simulink model "Main"  (R2021a)
settings: Solver=FixedStepDiscrete  StartTime=0.0  StopTime=3600  RelTol=1e-3  EnableMultiTasking=on
model workspace (MAT data in the model file):
  Rp_LUT = [0.0013213692114; 0.00132154036622; 0.00132170974574; 0.00132196270497; 0.00132238459891; 0.00132306078259; 0.001324076611; 0.00132551743918; 0.00132746862213; 0.00133001551485; 0.00133324347238; 0.00133723784971; 0.00134208400186; 0.00134786728385; 0.00135467305069; 0.00136258665738; 0.00137169345895; 0.0013820788104; 0.00139382806676; 0.00140702658302; 0.00142175971421; 0.00143811281533; 0.00145617124141; 0.00147602034745; 0.00149774548846; 0.00152143201947; 0.00154716529547; 0.00157503067149; 0.00160511350254; 0.00163749914362; 0.00167227294976; 0.00170952027597; 0.00174932647725]
  Rs_LUT = [0.00434482474387; 0.00419789131326; 0.00406794421213; 0.00395261023619; 0.00384993859762; 0.00375831094443; 0.00367637344064; 0.00360298484472; 0.00353717635596; 0.00347812023039; 0.00342510501023; 0.00337751579607; 0.00333481840341; 0.00329654653965; 0.00326229135038; 0.00323169283953; 0.0032044327828; 0.00318022883979; 0.00315882963473; 0.00314001062482; 0.00312357061298; 0.00310932879063; 0.00309712221887; 0.00308680367416; 0.00307823979817; 0.00307130950314; 0.00306590259229; 0.0030619185623; 0.00305926556038; 0.00305785947318; 0.00305762312844; 0.00305848559347; 0.00306038155708]
  ocv_LUT = [2.99933110368 3.09522958218 3.19229911251 3.28822862042 3.38021163392 3.46527495221 3.54075046741 3.60476472978 3.6565797805 3.69666389655 3.72648450624 3.74812569713 3.76387527119 3.77589456216 3.78601862589 3.79567838914 3.8059086629 3.81740274636 3.8305836234 3.84567360605 3.86275382653 3.88181106067 3.90277255901 3.92553086689 3.94996087864 3.97593115245 4.00331113101 4.03197552137 4.06180675196 4.09269615923 4.12454435791 4.15726110493 4.19076486521]
  soc_LUT = [0 0.03125 0.0625 0.09375 0.125 0.15625 0.1875 0.21875 0.25 0.28125 0.3125 0.34375 0.375 0.40625 0.4375 0.46875 0.5 0.53125 0.5625 0.59375 0.625 0.65625 0.6875 0.71875 0.75 0.78125 0.8125 0.84375 0.875 0.90625 0.9375 0.96875 1]
  tau_LUT = [1017.78463693; 1013.76600608; 1009.7449439; 1005.78640776; 1001.95428754; 998.311501769; 994.921511879; 991.866028712; 989.396935472; 988.873758798; 996.773296442; 1035.63338161; 1158.31056663; 1435.4479506; 1876.25610659; 2330.74386132; 2537.63289906; 2355.40456965; 1912.97681891; 1471.93759841; 1191.35445849; 1068.59098544; 1033.79837309; 1032.53037298; 1041.04700517; 1052.45769279; 1065.37076923; 1079.60983832; 1095.18901085; 1112.14336121; 1130.50876964; 1150.32016376; 1171.6114047]
values from neighbouring files (symbols this model uses):
  Ts = 0.2    [Parameters.m]
libraries: fl_lib x4, nesl_utility x4, ee_lib x1, sharedTrackingLibrary x1
settings Model: SimulationMode=accelerator  OrderedModelArguments=off  Creator=oscar  LastModifiedBy=oscar
settings SolverCC: AutoInsertRateTranBlk=on
settings DataIOCC: SaveOutput=off  SaveTime=off
settings OptimizationCC: DefaultParameterBehavior=Inlined  InlineInvariantSignals=on  EnhancedBackFolding=on  PassReuseOutputArgsAs=Individual arguments  StateBitsets=on  DataBitsets=on  ZeroExternalMemoryAtStartup=off  ZeroInternalMemoryAtStartup=off  NoFixptDivByZeroProtection=on  LifeSpan=1  OptimizeBlockOrder=speed  DifferentSizesBufferReuse=on  EfficientTunableParamExpr=on
settings DebuggingCC: ParameterTunabilityLossMsg=error
settings HardwareCC: ProdBitPerPointer=32  ProdBitPerSizeT=32  ProdBitPerPtrDiffT=32  ProdLargestAtomicInteger=Long  ProdLargestAtomicFloat=Double  ProdWordSize=32  ProdHWDeviceType=ARM Compatible->ARM Cortex-M
settings SFSimCC: MATLABDynamicMemAlloc=off
settings RTWCC: SystemTargetFile=ert.tlc  TLCOptions=-p0  GenCodeOnly=on  TemplateMakefile=ert_default_tmf  GenerateReport=on  RTWVerbose=off  IncludeHyperlinkInReport=on  LaunchReport=on
settings CodeAppCC: ForceParamTrailComments=on  IgnoreCustomStorageClasses=off  OperatorAnnotations=on  SimulinkDataObjDesc=on  SFDataObjDesc=on  CustomSymbolStrGlobalVar=rt$N$M  CustomSymbolStrType=$N$M  CustomSymbolStrFcn=$N$M$F  CustomSymbolStrMacro=$N$M  InsertBlockDesc=on
settings ERTTargetCC: TargetLangStandard=C99 (ISO)  CodeReplacementLibrary=ISO_C  GenerateSampleERTMain=on  IncludeMdlTerminateFcn=off  SuppressErrorStatus=on  SupportAbsoluteTime=off  SupportNonFinite=off  SupportComplex=off  InlinedParameterPlacement=NonHierarchical  RootIOFormat=Structure reference  ERTCustomFileTemplate=example_file_process.tlc
settings SimscapeCC: SimscapeLogType=all  SimscapeLogOpenViewer=on  SimscapeLogLimitData=off

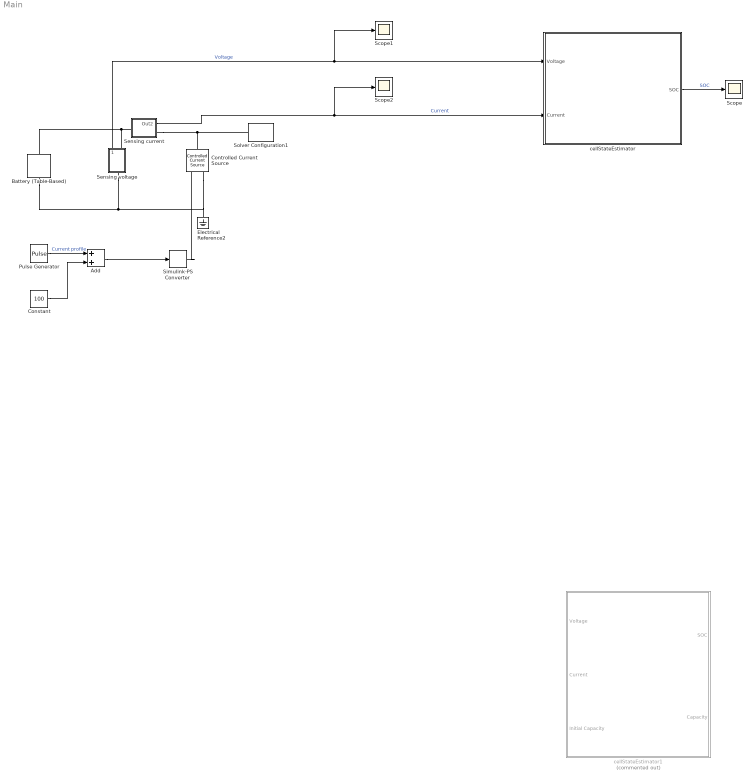
== system Main ==
  Add : Sum
  Battery (Table-Based) : ee_lib/Sources/Battery (Table-Based)  SOC_vec=soc_LUT  T_dependence=ee.enum.temperature_dependence.no  prm_dir=ee.enum.battery.prm_dir.noCurrentDirectionality  T_vec=[273.15, 298.15, 323.15] K  V0_mat=[3.2, 3.1, 3.14; 3.25, 3.27, 3.3; 3.28, 3.31, 3.34; 3.33, 3.5, 3.59] V  V0_vec=ocv_LUT V  R0_mat=[.03, .015, .002; .04, .017, .008; .039, .012, .006; .027, .013, .021] Ohm  R0_vec=Rs_LUT Ohm  R0_dis_mat=[.03, .015, .002; .04, .017, .008; .039, .012, .006; .027, .013, .021] Ohm  R0_dis_vec=[.015, .017, .012, .013] Ohm  R0_ch_mat=[.03, .015, .002; .04, .017, .008; .039, .012, .006; .027, .013, .021] Ohm  R0_ch_vec=[.015, .017, .012, .013] Ohm  AH_vec=[2.9, 4.1, 4.2] hr*A  AH=C hr*A  prm_leak=ee.enum.battery.prm_leak.disabled  Rleak_vec=[8000, 7000, 6000] Ohm  Rleak=7e3 Ohm  extrapolation_option=ee.enum.extrapolation.linear  prm_dyn=ee.enum.battery.prm_dyn.rc1  R1_mat=[.089, .076, .01; .042, .022, .099; .019, .007, .002; .051, .043, .029] Ohm  R1_vec=Rp_LUT Ohm  tau1_mat=[44, 148, 235; 93, 110, 1000; 19, 27, 133; .5, 22, 3] s  tau1_vec=tau_LUT s  R2_mat=[.014, .382, .407; .028, .006, .007; .014, .007, .006; .333, .956, .912] Ohm  R2_vec=[.382, .006, .007, .956] Ohm  tau2_mat=[1, 44, 5644; 11, 24, 506; 2, 14, 330; 3310, 13419, 30216] s  tau2_vec=[44, 24, 14, 13419] s  R3_mat=[.014, .382, .407; .028, .006, .007; .014, .007, .006; .333, .956, .912] Ohm  R3_vec=[.382, .006, .007, .956] Ohm  tau3_mat=[1, 44, 5644; 11, 24, 506; 2, 14, 330; 3310, 13419, 30216] s  tau3_vec=[44, 24, 14, 13419] s  R4_mat=[.014, .382, .407; .028, .006, .007; .014, .007, .006; .333, .956, .912] Ohm  R4_vec=[.382, .006, .007, .956] Ohm  tau4_mat=[1, 44, 5644; 11, 24, 506; 2, 14, 330; 3310, 13419, 30216] s  tau4_vec=[44, 24, 14, 13419] s  R5_mat=[.014, .382, .407; .028, .006, .007; .014, .007, .006; .333, .956, .912] Ohm  R5_vec=[.382, .006, .007, .956] Ohm  tau5_mat=[1, 44, 5644; 11, 24, 506; 2, 14, 330; 3310, 13419, 30216] s  tau5_vec=[44, 24, 14, 13419] s  prm_fade=ee.enum.battery.prm_fade.equations  N0=10  dV0=0  dR0=0  dAH=-2  dRleak=0  dR1=0  dR2=0  dR3=0  dR4=0  dR5=0  N0vec=[100, 200, 300]  Tfadevec=[298.15, 323.15] K  dV0vec=[0, 0, 0]  dR0vec=[0, 0, 0]  dAHvec=[0, 0, 0]  dRleakvec=[0, 0, 0]  dR1vec=[0, 0, 0]  dR2vec=[0, 0, 0]  dR3vec=[0, 0, 0]  dR4vec=[0, 0, 0]  dR5vec=[0, 0, 0]  dV0mat=[0, 0; 0, 0; 0, 0]  dR0mat=[0, 0; 0, 0; 0, 0]  dAHmat=[0, 0; 0, 0; 0, 0]  dRleakmat=[0, 0; 0, 0; 0, 0]  dR1mat=[0, 0; 0, 0; 0, 0]  dR2mat=[0, 0; 0, 0; 0, 0]  dR3mat=[0, 0; 0, 0; 0, 0]  dR4mat=[0, 0; 0, 0; 0, 0]  dR5mat=[0, 0; 0, 0; 0, 0]  prm_age=ee.enum.battery.prm_age.disabled  prm_age_OCV=ee.enum.battery.prm_age_OCV.OCV  OCV_age=0.9  SOC_age=0.6  storage_dt_age_vec=[0] d  storage_T_age_vec=[273] K  OCV_scaling_age=2.2134e6  OCV_offset_age=1.632e6  temp_exp_age=0.515833569 V  t_exp_age=0.75  T_age_vec=[273.15, 298.15, 323.15] K  dt_age_vec=[90, 180, 270, 360] d  dR0_age_vec=[0, 0, 0]  t_meas_dR0_age=100 d  dR0_age_mat=[0, 0, 0; 0, 0, 0; 0, 0, 0; 0, 0, 0]  temperature=298.15 K  i_specify=off  i_priority=None  i=0 A  i_nominal_specify=off  i_nominal_unit=A  i_nominal_value=1  v_specify=off  v_priority=None  v=0 V  v_nominal_specify=off  v_nominal_unit=V  v_nominal_value=1  stateOfCharge_specify=on  stateOfCharge_priority=High  stateOfCharge=0.7  stateOfCharge_nominal_specify=off  stateOfCharge_nominal_unit=1  stateOfCharge_nominal_value=1  num_cycles_specify=off  num_cycles_priority=High  num_cycles=0  num_cycles_nominal_specify=off  num_cycles_nominal_unit=1  num_cycles_nominal_value=1  thermal_mass=30000 J/K  temperature_specify=off  temperature_priority=High  temperature_nominal_specify=off  temperature_nominal_unit=K  temperature_nominal_value=1
      settings: SourceProductBaseCode=PS  InternalSimscapePortConfiguration="{\"Bottom\":[],\"Left\":[{\"id\":\"p\",\"label\":\"+\",\"type\":\"foundation.electrical.electrical\"}],\"Right\":[{\"id\":\"n\",\"label\":\"-\",\"type\":\"foundation.electrical.electrical\"}],\"Top\":[]}"
  Constant : Constant  Value=100
  Controlled Current Source : fl_lib/Electrical/Electrical Sources/Controlled Current Source
  Electrical Reference2 : fl_lib/Electrical/Electrical Elements/Electrical Reference
  Pulse Generator : DiscretePulseGenerator  Amplitude=-200  Period=30/0.2  PulseWidth=0.5*30/0.2  SampleTime=0.2
  Scope : Scope
  Scope1 : Scope
  Scope2 : Scope
  Sensing current : Subsystem
      mask Display: disp('i')
  Sensing voltage : Subsystem
      mask Display: disp('i')
  Simulink-PS Converter : nesl_utility/Simulink-PS Converter  PhysicalDomain=network_engine_domain  SubClassName=ps_input  LeftPortType=input  RightPortType=output  PseudoPeriodic=off  Frequencies=[]  NoiseDistribution=none  NoiseParameters=[]  Unit=A  AffineConversion=off  FilteringAndDerivatives=zero  SimscapeFilterOrder=1  InputFilterTimeConstant=0.001  UdotUserProvided=1
      settings: SourceProductBaseCode=PW,SS
  Solver Configuration1 : nesl_utility/Solver Configuration  PhysicalDomain=network_engine_domain  SubClassName=solver  LeftPortType=input  RightPortType=generic  Tones=[]  Harmonics=[]  SimulateNoise=off  Profile=off  UseLocalSampling=off  EnableSwitchedLinearOptims=on  FrequencyDomain=off  UseCCode=off  RelTol=0.001  AbsTol=1e-06  MinStep=1e-09  ToWorkspace=off  RevertToSquareIcSolve=off  NumHomotopyIterations=100  PhasorMode=off  PhasorModeNumHarmonics=1  DoDC=off  ResidualTolerance=1e-09  UseLocalSolver=on  LocalSolverChoice=NE_BACKWARD_EULER_ADVANCER  LocalSolverSampleTime=Ts  DoFixedCost=on  MaxNonlinIter=3  MaxModeIter=2  ComputeImpulses=off  ImpulseIterations=2  LinearAlgebra=auto  EquationFormulation=NE_TIME_EF  DelaysMemoryBudget=1024  AutomaticFiltering=on  FilteringTimeConstant=0.001  PartitionStorageMethod=AS_NEEDED  PartitionMemoryBudget=1024  PartitionMethod=FAST
      settings: SourceProductBaseCode=PW,SS
  cellStateEstimator : Subsystem
  cellStateEstimator1 : Subsystem  Commented=on
  wires:
  cellStateEstimator/1(SOC) -> Scope/1  "SOC"
  Sensing voltage/1(Out1) -> Scope1/1, cellStateEstimator/1(Voltage)  "Voltage"
  Pulse Generator/1 -> Add/1  "Current profile"
  Sensing current/1(Out2) -> Scope2/1, cellStateEstimator/2(Current)  "Current"
  Constant/1 -> Add/2
  Add/1 -> Simulink-PS Converter/1
  connections:
  Sensing voltage/RConn1 -- Battery (Table-Based)/LConn1 -- Sensing current/LConn1
  Solver Configuration1/RConn1 -- Sensing current/RConn1 -- Controlled Current Source/LConn1
  Electrical Reference2/LConn1 -- Controlled Current Source/RConn2 -- Battery (Table-Based)/RConn1 -- Sensing voltage/LConn1
  Simulink-PS Converter/RConn1 -- Controlled Current Source/RConn1

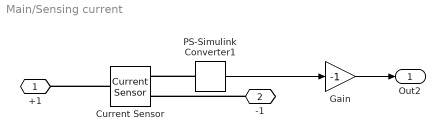
== system Main/Sensing current ==
  Current Sensor : fl_lib/Electrical/Electrical Sensors/Current Sensor
  Gain : Gain  Gain=-1
  PS-Simulink Converter1 : nesl_utility/PS-Simulink Converter  PhysicalDomain=network_engine_domain  SubClassName=ps_output  LeftPortType=input  RightPortType=output  PseudoPeriodic=off  Frequencies=[]  Unit=A  AffineConversion=off
      settings: SourceProductBaseCode=PW,SS
  +1 : PMIOPort  Side=Left
  -1 : PMIOPort  Port=2  Side=Right
  Out2 : Outport  VectorParamsAs1DForOutWhenUnconnected=off
  wires:
  Gain/1 -> Out2/1
  PS-Simulink Converter1/1 -> Gain/1
  connections:
  -1/RConn1 -- Current Sensor/RConn2
  PS-Simulink Converter1/LConn1 -- Current Sensor/RConn1
  Current Sensor/LConn1 -- +1/RConn1

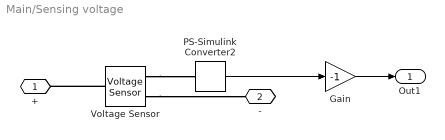
== system Main/Sensing voltage ==
  Gain : Gain  Gain=-1
  PS-Simulink Converter2 : nesl_utility/PS-Simulink Converter  PhysicalDomain=network_engine_domain  SubClassName=ps_output  LeftPortType=input  RightPortType=output  PseudoPeriodic=off  Frequencies=[]  Unit=V  AffineConversion=off
      settings: SourceProductBaseCode=PW,SS
  Voltage Sensor : fl_lib/Electrical/Electrical Sensors/Voltage Sensor
  + : PMIOPort  Side=Left
  - : PMIOPort  Port=2  Side=Right
  Out1 : Outport  VectorParamsAs1DForOutWhenUnconnected=off
  wires:
  PS-Simulink Converter2/1 -> Gain/1
  Gain/1 -> Out1/1
  connections:
  Voltage Sensor/RConn2 -- -/RConn1
  Voltage Sensor/RConn1 -- PS-Simulink Converter2/LConn1
  Voltage Sensor/LConn1 -- +/RConn1

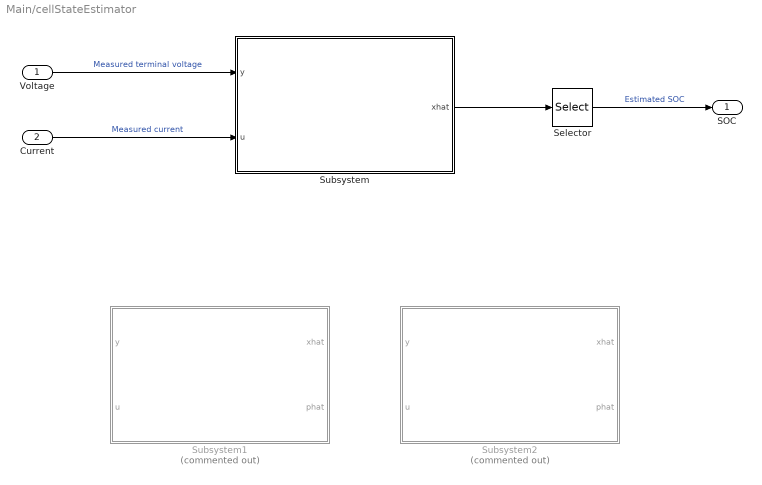
== system Main/cellStateEstimator ==
  Voltage : Inport
  Current : Inport  Port=2
  Selector : Selector  InputPortWidth=2  IndexOptions=Index vector (dialog)  Indices=[2]  OutputSizes=1
  Subsystem : Subsystem
  Subsystem1 : Subsystem  Commented=on
  Subsystem2 : Subsystem  Commented=on
  SOC : Outport
  wires:
  Selector/1 -> SOC/1  "Estimated SOC"
  Current/1 -> Subsystem/2(u)  "Measured current"
  Voltage/1 -> Subsystem/1(y)  "Measured terminal voltage"
  Subsystem/1(xhat) -> Selector/1

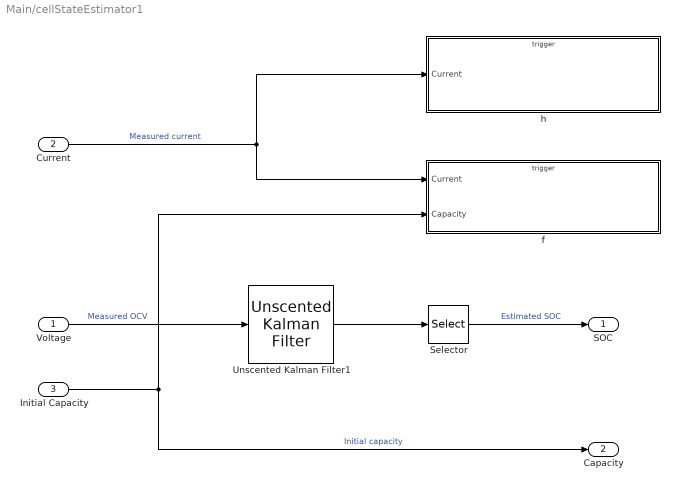
== system Main/cellStateEstimator1 ==
  Voltage : Inport
  Current : Inport  Port=2
  Initial Capacity : Inport  Port=3
  Selector : Selector  InputPortWidth=2  IndexOptions=Index vector (dialog)  Indices=[1]  OutputSizes=1
  Unscented Kalman Filter1 : sharedTrackingLibrary/Unscented Kalman Filter  StateTransitionFcn=batteryStateFcn  HasAdditiveProcessNoise=Additive  ProcessNoise=Q0  HasTimeVaryingProcessNoise=off  HasStateTransitionFcnExtraArgument=0  InitialState=x0  InitialStateCovariance=P0  Alpha=1  Beta=2  Kappa=0  MeasurementFcn1=batteryMeasurementFcn  HasMeasurementEnablePort1=off  HasAdditiveMeasurementNoise1=Additive  MeasurementNoise1=R0  HasTimeVaryingMeasurementNoise1=off  HasMeasurementFcnExtraArgument1=0  MeasurementFcn2=myMeasurementFcn  HasMeasurementEnablePort2=off  HasAdditiveMeasurementNoise2=Additive  MeasurementNoise2=1  HasTimeVaryingMeasurementNoise2=off  HasMeasurementFcnExtraArgument2=0  MeasurementFcn3=myMeasurementFcn  HasMeasurementEnablePort3=off  HasAdditiveMeasurementNoise3=Additive  MeasurementNoise3=1  HasTimeVaryingMeasurementNoise3=off  HasMeasurementFcnExtraArgument3=0  MeasurementFcn4=myMeasurementFcn  HasMeasurementEnablePort4=off  HasAdditiveMeasurementNoise4=Additive  MeasurementNoise4=1  HasTimeVaryingMeasurementNoise4=off  HasMeasurementFcnExtraArgument4=0  MeasurementFcn5=myMeasurementFcn  HasMeasurementEnablePort5=off  HasAdditiveMeasurementNoise5=Additive  MeasurementNoise5=1  HasTimeVaryingMeasurementNoise5=off  HasMeasurementFcnExtraArgument5=0  EnableMultirate=off  StateTransitionFcnSampleTime=1  MeasurementFcn1SampleTime=1  MeasurementFcn2SampleTime=1  MeasurementFcn3SampleTime=1  MeasurementFcn4SampleTime=1  MeasurementFcn5SampleTime=1  UseCurrentEstimator=on  OutputStateCovariance=off  DataType=double  SampleTime=Ts  NumberOfMeasurements=1
      settings: SourceProductBaseCode=CT,DR,TF,ID,LP,NV,AR,RO,RR,UV,VE
  f : Subsystem  TreatAsAtomicUnit=on
  h : Subsystem  TreatAsAtomicUnit=on
  SOC : Outport
  Capacity : Outport  Port=2
  wires:
  Selector/1 -> SOC/1  "Estimated SOC"
  Current/1 -> f/1(Current), h/1(Current)  "Measured current"
  Voltage/1 -> Unscented Kalman Filter1/1  "Measured OCV"
  Unscented Kalman Filter1/1 -> Selector/1
  Initial Capacity/1 -> f/2(Capacity), Capacity/1  "Initial capacity"

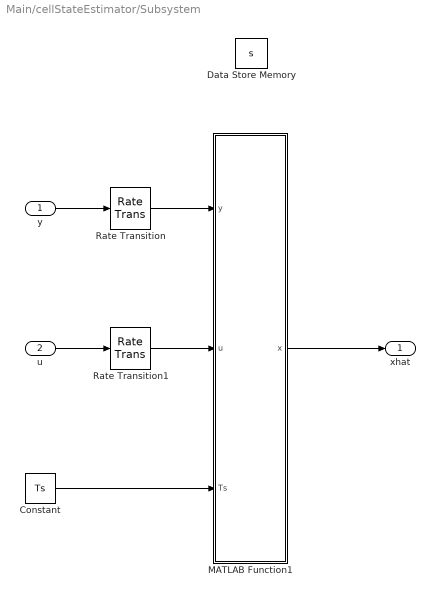
== system Main/cellStateEstimator/Subsystem ==
  y : Inport
  u : Inport  Port=2
  Constant : Constant  Value=Ts
  Data Store Memory : DataStoreMemory  DataStoreName=s  ReadBeforeWriteMsg=warning  WriteAfterWriteMsg=warning  WriteAfterReadMsg=warning  InitialValue=s0  ShowAdditionalParam=off  OutDataTypeStr=Bus: AF_state
  MATLAB Function1 : MATLAB Function  TreatAsAtomicUnit=on
  Rate Transition : RateTransition  OutPortSampleTime=Ts
  Rate Transition1 : RateTransition  OutPortSampleTime=Ts
  xhat : Outport
  wires:
  y/1 -> Rate Transition/1
  Constant/1 -> MATLAB Function1/3(Ts)
  Rate Transition/1 -> MATLAB Function1/1(y)
  u/1 -> Rate Transition1/1
  Rate Transition1/1 -> MATLAB Function1/2(u)
  MATLAB Function1/1(x) -> xhat/1

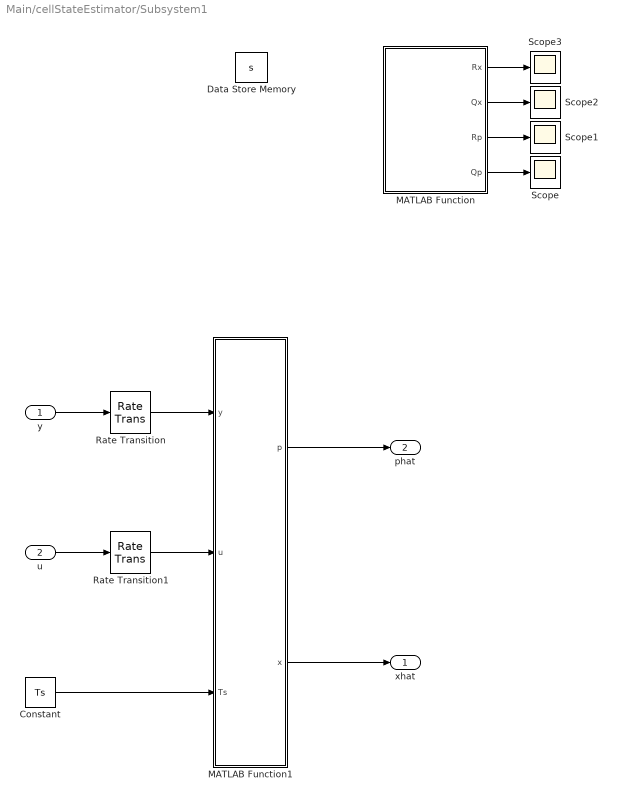
== system Main/cellStateEstimator/Subsystem1 ==
  y : Inport
  u : Inport  Port=2
  Constant : Constant  Value=Ts
  Data Store Memory : DataStoreMemory  DataStoreName=s  ReadBeforeWriteMsg=warning  WriteAfterWriteMsg=warning  WriteAfterReadMsg=warning  InitialValue=s0  ShowAdditionalParam=off  OutDataTypeStr=Bus: MAF_state
  MATLAB Function : MATLAB Function  TreatAsAtomicUnit=on
  MATLAB Function1 : MATLAB Function  TreatAsAtomicUnit=on
  Rate Transition : RateTransition  OutPortSampleTime=Ts
  Rate Transition1 : RateTransition  OutPortSampleTime=Ts
  Scope{,1..3} (4 alike) : Scope
  xhat : Outport
  phat : Outport  Port=2
  wires:
  y/1 -> Rate Transition/1
  Constant/1 -> MATLAB Function1/3(Ts)
  Rate Transition/1 -> MATLAB Function1/1(y)
  u/1 -> Rate Transition1/1
  Rate Transition1/1 -> MATLAB Function1/2(u)
  MATLAB Function1/2(x) -> xhat/1
  MATLAB Function1/1(p) -> phat/1
  MATLAB Function/4(Qp) -> Scope/1
  MATLAB Function/3(Rp) -> Scope1/1
  MATLAB Function/2(Qx) -> Scope2/1
  MATLAB Function/1(Rx) -> Scope3/1

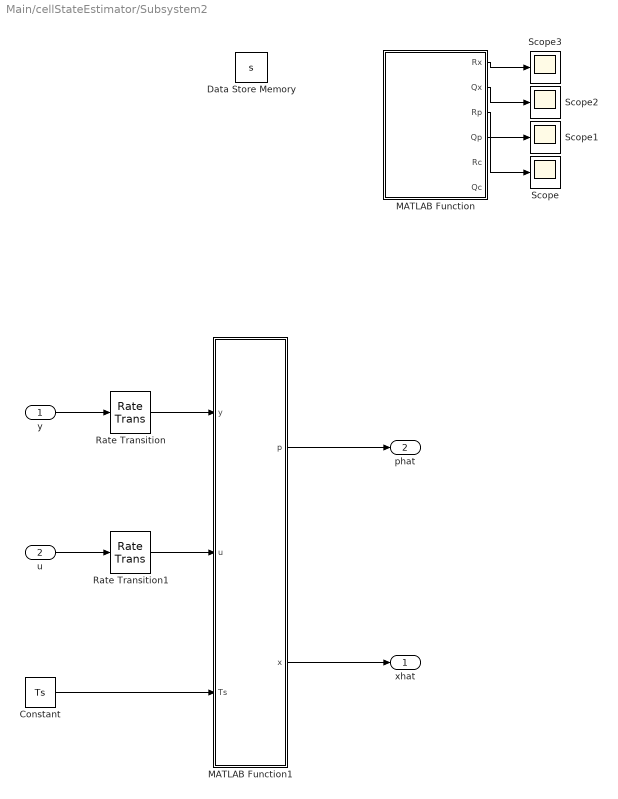
== system Main/cellStateEstimator/Subsystem2 ==
  y : Inport
  u : Inport  Port=2
  Constant : Constant  Value=Ts
  Data Store Memory : DataStoreMemory  DataStoreName=s  ReadBeforeWriteMsg=warning  WriteAfterWriteMsg=warning  WriteAfterReadMsg=warning  InitialValue=s0  ShowAdditionalParam=off  OutDataTypeStr=Bus: MAF_state
  MATLAB Function : MATLAB Function  TreatAsAtomicUnit=on
  MATLAB Function1 : MATLAB Function  TreatAsAtomicUnit=on
  Rate Transition : RateTransition  OutPortSampleTime=Ts
  Rate Transition1 : RateTransition  OutPortSampleTime=Ts
  Scope{,1..3} (4 alike) : Scope
  xhat : Outport
  phat : Outport  Port=2
  wires:
  y/1 -> Rate Transition/1
  Constant/1 -> MATLAB Function1/3(Ts)
  Rate Transition/1 -> MATLAB Function1/1(y)
  u/1 -> Rate Transition1/1
  Rate Transition1/1 -> MATLAB Function1/2(u)
  MATLAB Function1/2(x) -> xhat/1
  MATLAB Function1/1(p) -> phat/1
  MATLAB Function/4(Qp) -> Scope/1
  MATLAB Function/3(Rp) -> Scope1/1
  MATLAB Function/2(Qx) -> Scope2/1
  MATLAB Function/1(Rx) -> Scope3/1

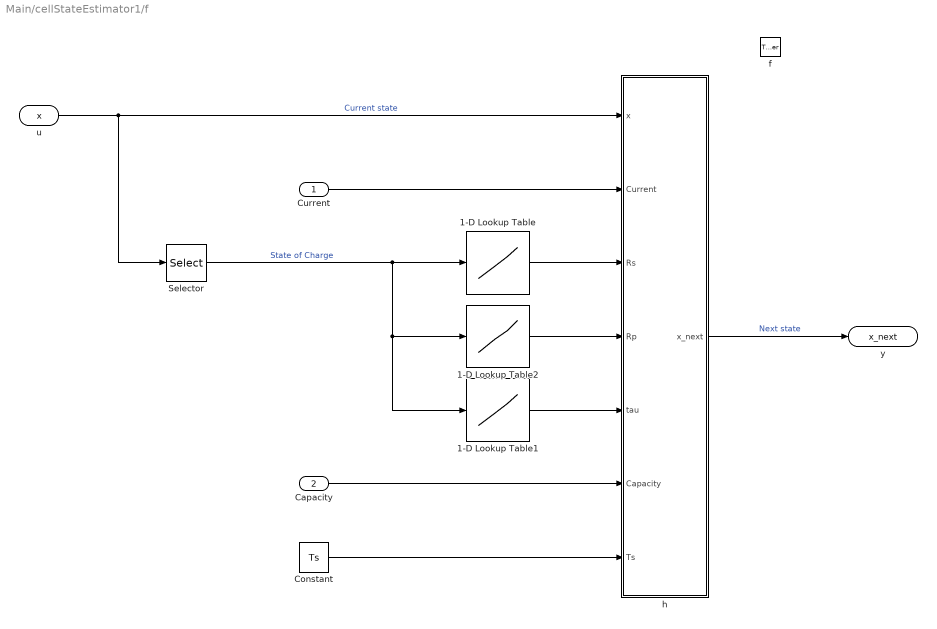
== system Main/cellStateEstimator1/f ==
  Current : Inport
  Capacity : Inport  Port=2
  f : TriggerPort  TriggerType=function-call  IsSimulinkFunction=on  FunctionName=batteryStateFcn  FunctionVisibility=scoped  VariantControl=(inherit)
  1-D Lookup Table : Lookup_n-D  NumberOfTableDimensions=1  BreakpointsForDimension1=soc_LUT  Table=Rs_LUT  InternalRulePriority=Speed  RndMeth=Simplest  InputSameDT=on
  1-D Lookup Table1 : Lookup_n-D  NumberOfTableDimensions=1  BreakpointsForDimension1=soc_LUT  Table=tau_LUT  InternalRulePriority=Speed  RndMeth=Simplest  InputSameDT=on
  1-D Lookup Table2 : Lookup_n-D  NumberOfTableDimensions=1  BreakpointsForDimension1=soc_LUT  Table=Rp_LUT  InternalRulePriority=Speed  RndMeth=Simplest  InputSameDT=on
  Constant : Constant  Value=Ts
  Selector : Selector  InputPortWidth=2  IndexOptions=Index vector (dialog)  Indices=[1]  OutputSizes=1
  h : MATLAB Function  TreatAsAtomicUnit=on
  u : ArgIn  DisableCoverage=on  PortDimensions=2  ArgumentName=x
  y : ArgOut  DisableCoverage=on  PortDimensions=2  ArgumentName=x_next
  wires:
  u/1 -> h/1(x), Selector/1  "Current state"
  Selector/1 -> 1-D Lookup Table2/1, 1-D Lookup Table1/1, 1-D Lookup Table/1  "State of Charge"
  1-D Lookup Table/1 -> h/3(Rs)
  1-D Lookup Table1/1 -> h/5(tau)
  Current/1 -> h/2(Current)
  Capacity/1 -> h/6(Capacity)
  h/1(x_next) -> y/1  "Next state"
  Constant/1 -> h/7(Ts)
  1-D Lookup Table2/1 -> h/4(Rp)

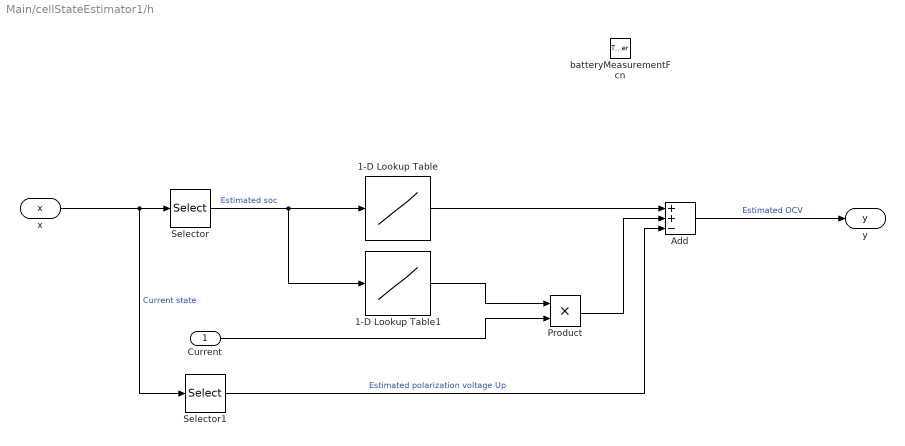
== system Main/cellStateEstimator1/h ==
  Current : Inport
  batteryMeasurementFcn : TriggerPort  TriggerType=function-call  IsSimulinkFunction=on  FunctionName=batteryMeasurementFcn  FunctionVisibility=scoped  VariantControl=(inherit)
  1-D Lookup Table : Lookup_n-D  NumberOfTableDimensions=1  BreakpointsForDimension1=soc_LUT  Table=ocv_LUT  InternalRulePriority=Speed  RndMeth=Simplest  InputSameDT=on
  1-D Lookup Table1 : Lookup_n-D  NumberOfTableDimensions=1  BreakpointsForDimension1=soc_LUT  Table=Rs_LUT  InternalRulePriority=Speed  RndMeth=Simplest  InputSameDT=on
  Add : Sum  Inputs=++-
  Product : Product
  Selector : Selector  InputPortWidth=2  IndexOptions=Index vector (dialog)  Indices=[1]  OutputSizes=1
  Selector1 : Selector  InputPortWidth=2  IndexOptions=Index vector (dialog)  Indices=[2]  OutputSizes=1
  x : ArgIn  DisableCoverage=on  PortDimensions=2  ArgumentName=x
  y : ArgOut  DisableCoverage=on  ArgumentName=y
  wires:
  x/1 -> Selector1/1, Selector/1  "Current state"
  Selector/1 -> 1-D Lookup Table/1, 1-D Lookup Table1/1  "Estimated soc"
  1-D Lookup Table/1 -> Add/1
  1-D Lookup Table1/1 -> Product/1
  Current/1 -> Product/2
  Product/1 -> Add/2
  Selector1/1 -> Add/3  "Estimated polarization voltage Up"
  Add/1 -> y/1  "Estimated OCV"

== matlab function Main/cellStateEstimator1/f/h ==
  data: x input; Current input; x_next output; Rs input; Rp input; tau input; Capacity input; Ts input
% @brief    The state transistion function. Check page 120 in in Xiong BMS 2020
% @param    The current state x = [ soc, Up ]' (state of charge, also
%           denoted z, and the polarizaton voltage Up)
% @param    The current running through the battery. Positive sign
%           indicates current draw (soc is reduced when current is drawn).
% @param    The equivalent series resistance
% @param    The equivalent polarisation resistance
% @param    The equivalent polarisation capacitance
% @param    The total capacity of the cell. (C-rating times 3600)
% @param    The sampling frequency of the system (time-step length)
% @retval   The next state, x = [ soc, Up ]'
function x_next = f(x, Current, Rs, Rp, tau, Capacity, Ts)
x_next = zeros(2, 1);


x_next(1) = x(1) - Ts * Current / Capacity;
x_next(2) = exp(-Ts / tau) * x(2) - (1 - exp(-Ts / tau)) * Rp * Current;
end

== matlab function Main/cellStateEstimator/Subsystem1/MATLAB Function ==
  data: Rx output; Qx output; Rp output; Qp output; s data_store_memory
function [Rx, Qx, Rp, Qp] = display_stats

global s;

Rx = s.Rx;
Qx = s.Qx;
Rp = s.Rp;
Qp = s.Qp;

end

== matlab function Main/cellStateEstimator/Subsystem1/MATLAB Function1 ==
  data: p output; y input; u input; Ts input; x output; s data_store_memory
function [p, x] = MAF(y, u, Ts)

global s;

%% MAEKF state correction
AEKF_state_correction(y, u, Ts);

%% this is how multi-timescale is implemented
s.k = uint16(mod(s.k + 1, s.K) + 1);
if s.k == 6
    %% MAEKF parameter correction
    AEKF_parameter_correction(y, u, Ts);
    
    %% MAEKF parameter prediction
    AEKF_parameter_prediction(y, u, Ts);
end

%% MAEKF state prediction last
AEKF_state_prediction(y, u, Ts);

x = s.x_;
p = s.p_;

end

%% State Correction

function AEKF_state_correction(y, u, Ts)

global s;

Cx = Cx_Fcn(s.x_, s.p_, u, Ts);

Ex = y - h(s.x_, s.p_, u, Ts);
Kx = s.Px_ * Cx' * inv(Cx * s.Px_ * Cx' + s.Rx);
s.x = s.x_ + Kx * Ex;
KCx = Kx * Cx;
s.Px = (eye(size(KCx)) - KCx) * s.Px_;

Hx = cov(s.Ex);

s.lx = uint16(mod(s.lx + 1, s.Lx) + 1);
s.Ex(s.lx) = Ex;

aRx = Hx + Cx * s.Px * Cx';
%rx = exp(-abs(aRx - s.Rx));
rx = 0.95;
s.Rx = rx * s.Rx + (1 - rx) * aRx;

aQx = Kx * Hx * Kx';
%qx = exp(-abs(aQx - s.Qx));
qx = 0.95;
s.Qx = qx * s.Qx + (1 - qx) * aQx;

end

%% State Prediction

function AEKF_state_prediction(y, u, Ts)

global s

Ax = Ax_Fcn(s.x, s.p_, u, Ts);

s.x_ = f(s.x, s.p_, u, Ts);
s.Px_ = Ax * s.Px * Ax' + s.Qx;

end

%% Parameter Correction

function AEKF_parameter_correction(y, u, Ts)

global s;

Cp = Cp_Fcn(s.x, y, s.p_, u, Ts);

Ep = y - h(s.x, s.p_, u, Ts);
Kp = s.Pp_ * Cp' * inv(Cp * s.Pp_ * Cp' + s.Rp);
s.p = s.p_ + Kp * Ep;
KCp = Kp * Cp;
s.Pp = (eye(size(KCp)) - KCp) * s.Pp_;

Hp = cov(s.Ep);

s.lp = uint16(mod(s.lp + 1, s.Lp) + 1);
s.Ep(s.lp) = Ep;

aRp = Hp + Cp * s.Pp * Cp';
%rp = exp(-abs(aRp - s.Rp));
rp = 0.95;
s.Rp = rp * s.Rp + (1 - rp) * aRp;

aQp = Kp * Hp * Kp';
%qp = exp(-abs(aQp - s.Qp));
qp = 0.95;
s.Qp = qp * s.Qp + (1 - qp) * aQp;
end

%% Parameter Prediction

function AEKF_parameter_prediction(y, u, Ts)

global s

s.p_ = s.p;
s.Pp_ = s.Pp + s.Qp;

end

%% OCV and it's derivative with respect to soc (denoted z)

function ocv = ocv_Fcn(z)
g = [-5.90241040764213,13.2176608408928,-6.67518652537707,-2.97531430827542,3.52891506032032,2.99808472821531];

ocv = g(1)*z.^5 + g(2)*z.^4 + g(3)*z.^3 + g(4)*z.^2 + g(5)*z.^1 + g(6);
end

function soc = soc_Fcn(x)
g = [0.502188960650572,-8.22345027526894,53.6697762791713,-174.553359527449,283.022401329238,-183.103467383057];
w = [-10.5849149607721,37.0498014971184,-42.7964981127015];

soc = (g(1)*x.^5 + g(2)*x.^4 + g(3)*x.^3 + g(4)*x.^2 + g(5)*x.^1 + g(6)) ./ (x.^3 + w(1)*x.^2 + w(2)*x.^1 + w(3));
end

function docv = docv_Fcn(z)
g = [-5.90241040764213,13.2176608408928,-6.67518652537707,-2.97531430827542,3.52891506032032,2.99808472821531];

docv = g(1)*z.^4 + g(2)*z.^3 + g(3)*z.^2 + g(4)*z.^1 + g(5);
end

%% A, B, C, D state matrices

function Ax = Ax_Fcn(x, p, u, Ts)
Ax = [ 
    exp(-Ts / p(3)), 0;
    0, 1
];
end

function Bx = Bx_Fcn(x, p, u, Ts)
Bx = [ 
    (1 - exp(-Ts / p(3))) * p(2);
    Ts / p(4)
];
end

function Cx = Cx_Fcn(x, p, u, Ts)
Cx = [ -1,  docv_Fcn(x(2)) ];
end

function Dx = Dx_Fcn(x, p, u, Ts)
Dx = ocv_Fcn(x(2)) - u * p(1) - x(1) - Cx_Fcn(x, p, u, Ts) * x;
end

%% C parameter matrix

function Cp = Cp_Fcn(x, y, p, u, Ts)

Cx = Cx_Fcn(x, p, u, Ts);
Ax = Ax_Fcn(x, p, u, Ts);

dfdp12 =  -u * (exp(-Ts / p(3)) - 1);
dfdp13 =  -(u * p(2) - x(1)) * Ts * exp(-Ts / p(3)) / p(3)^2;
dfdp24 =  u * Ts / p(4)^2;

dfdp = [ 
    0, dfdp12, dfdp13, 0;
    0, 0, 0, dfdp24
];

Cp1 = [ -u, 0, 0, docv_Fcn(x(1)) * u * Ts / p(4)^2 ];
Cp2 = Cx*(dfdp + Ax*dxdp);
Cp = Cp1 + Cp2;

end

%% Capacity C matrix

function Cc = Cc_Fcn(x, p, u, Ts)

Cc = docv_Fcn(x(1)) * u * Ts / p(4)^2;

end

%% the F (state transition) and H (measurement) functions

function x_next = f(x, p, u, Ts)
x_next = Ax_Fcn(x, p, u, Ts) * x + Bx_Fcn(x, p, u, Ts) * u;
end

function y = h(x, p, u, Ts)
y = ocv_Fcn(x(2)) - u * p(1) - x(1);
end

== matlab function Main/cellStateEstimator/Subsystem2/MATLAB Function ==
  data: Rx output; Qx output; Rp output; Qp output; s data_store_memory; Rc output; Qc output
function [Rx, Qx, Rp, Qp, Rc, Qc] = display_stats

global s;

Rx = s.Rx;
Qx = s.Qx;
Rp = s.Rp;
Qp = s.Qp;
Rc = s.Rc;
Qc = s.Qc;

end

== matlab function Main/cellStateEstimator/Subsystem2/MATLAB Function1 ==
  data: p output; y input; u input; Ts input; x output; s data_store_memory
function [p, x] = MAF(y, u, Ts)

global s;

%% MAEKF state correction
AEKF_state_correction(y, u, Ts);

%% this is how multi-timescale is implemented
s.k = uint16(mod(s.k + 1, s.K) + 1);
if s.k == 6
    %% MAEKF parameter correction
    AEKF_parameter_correction(y, u, Ts);
    
    %% MAEKF parameter prediction
    AEKF_parameter_prediction(y, u, Ts);
end

%% MAEKF state prediction last
AEKF_state_prediction(y, u, Ts);

x = s.x_;
p = s.p_;

end

%% State Correction

function AEKF_state_correction(y, u, Ts)

global s;

Cx = Cx_Fcn(s.x_, s.p_, u, Ts);

Ex = y - h(s.x_, s.p_, u, Ts);
Kx = s.Px_ * Cx' * inv(Cx * s.Px_ * Cx' + s.Rx);
s.x = s.x_ + Kx * Ex;
KCx = Kx * Cx;
s.Px = (eye(size(KCx)) - KCx) * s.Px_;

Hx = cov(s.Ex);

s.lx = uint16(mod(s.lx + 1, s.Lx) + 1);
s.Ex(s.lx) = Ex;

aRx = Hx + Cx * s.Px * Cx';
%rx = exp(-abs(aRx - s.Rx));
rx = 0.95;
s.Rx = rx * s.Rx + (1 - rx) * aRx;

aQx = Kx * Hx * Kx';
%qx = exp(-abs(aQx - s.Qx));
qx = 0.95;
s.Qx = qx * s.Qx + (1 - qx) * aQx;

end

%% State Prediction

function AEKF_state_prediction(y, u, Ts)

global s

Ax = Ax_Fcn(s.x, s.p_, u, Ts);

s.x_ = f(s.x, s.p_, u, Ts);
s.Px_ = Ax * s.Px * Ax' + s.Qx;

end

%% Parameter Correction

function AEKF_parameter_correction(y, u, Ts)

global s;

Cc = Cp_Fcn(s.x, y, s.p_, u, Ts);

Ep = y - h(s.x, s.p_, u, Ts);
Kc = s.Pc_ * Cc' * inv(Cc * s.Pc_ * Cc' + s.Rc);
s.c = s.c_ + Kc * Ep;
KCc = Kc * Cc;
s.Pc = (eye(size(KCc)) - KCc) * s.Pc_;
s.p(4) = s.c;

Hc = cov(s.Ep);

s.lc = uint16(mod(s.lc + 1, s.Lc) + 1);
s.Ep(s.lc) = Ep;

aRc = Hc + Cc * s.Pc * Cc';
rc = 0.95;
s.Rc = rc * s.Rc + (1 - rc) * aRc;

aQc = Kc * Hc * Kc';
qc = 0.95;
s.Qc = qc * s.Qc + (1 - qc) * aQc;

end

%% Parameter Prediction

function AEKF_parameter_prediction(y, u, Ts)

global s

s.c_ = s.c;
s.p_ = s.p;
s.Pc_ = s.Pc + s.Qc;

end

%% OCV and it's derivative with respect to soc (denoted z)

function ocv = ocv_Fcn(z)
g = [-5.90241040764213,13.2176608408928,-6.67518652537707,-2.97531430827542,3.52891506032032,2.99808472821531];

ocv = g(1)*z.^5 + g(2)*z.^4 + g(3)*z.^3 + g(4)*z.^2 + g(5)*z.^1 + g(6);
end

function soc = soc_Fcn(x)
g = [0.502188960650572,-8.22345027526894,53.6697762791713,-174.553359527449,283.022401329238,-183.103467383057];
w = [-10.5849149607721,37.0498014971184,-42.7964981127015];

soc = (g(1)*x.^5 + g(2)*x.^4 + g(3)*x.^3 + g(4)*x.^2 + g(5)*x.^1 + g(6)) ./ (x.^3 + w(1)*x.^2 + w(2)*x.^1 + w(3));
end

function docv = docv_Fcn(z)
g = [-5.90241040764213,13.2176608408928,-6.67518652537707,-2.97531430827542,3.52891506032032,2.99808472821531];

docv = g(1)*z.^4 + g(2)*z.^3 + g(3)*z.^2 + g(4)*z.^1 + g(5);
end

%% A, B, C, D state matrices

function Ax = Ax_Fcn(x, p, u, Ts)
Ax = [ 
    exp(-Ts / p(3)), 0;
    0, 1
];
end

function Bx = Bx_Fcn(x, p, u, Ts)
Bx = [ 
    (1 - exp(-Ts / p(3))) * p(2);
    Ts / p(4)
];
end

function Cx = Cx_Fcn(x, p, u, Ts)
Cx = [ -1,  docv_Fcn(x(2)) ];
end

function Dx = Dx_Fcn(x, p, u, Ts)
Dx = ocv_Fcn(x(2)) - u * p(1) - x(1) - Cx_Fcn(x, p, u, Ts) * x;
end

%% C parameter matrix

function x = x_of_p(p, y, u, Ts)

global s

Cx = Cx_Fcn(s.x_, p, u, Ts);

Ex = y - h(s.x_, p, u, Ts);
Kx = s.Px_ * Cx' * inv(Cx * s.Px_ * Cx' + s.Rx);

x = s.x_ + Kx * Ex;

end

function Cp = Cp_Fcn(x, y, p, u, Ts)

Cx = Cx_Fcn(x, p, u, Ts);
Ax = Ax_Fcn(x, p, u, Ts);

dfdp12 =  u * (exp(-Ts / p(3)) - 1);
dfdp13 =  (u * p(2) - x(1)) * Ts * exp(-Ts / p(3)) / p(3)^2;
dfdp24 =  u * Ts / p(4)^2;

dfdp = [ 
    0, dfdp12, dfdp13, 0;
    0, 0, 0, dfdp24
];

e = 0.01;
dp1 = [ e * p(1), 0, 0, 0 ]';
dp2 = [ 0, e * p(2), 0, 0 ]';
dp3 = [ 0, 0, e * p(3), 0 ]';
dp4 = [ 0, 0, 0, e * p(4) ]';

dxdp1 = (f(x, p + dp1, u, Ts) - f(x, p - dp1, u, Ts)) / norm(2*dp1);
dxdp2 = (f(x, p + dp2, u, Ts) - f(x, p - dp2, u, Ts)) / norm(2*dp2);
dxdp3 = (f(x, p + dp3, u, Ts) - f(x, p - dp3, u, Ts)) / norm(2*dp3);
dxdp4 = (f(x, p + dp4, u, Ts) - f(x, p - dp4, u, Ts)) / norm(2*dp4);


dxdp = [ dxdp1, dxdp2, dxdp3, dxdp4 ];
Cp = dfdp24 * docv_Fcn(x(2)) + Cx * dxdp4;

end


%% the F (state transition) and H (measurement) functions

function x_next = f(x, p, u, Ts)
x_next = Ax_Fcn(x, p, u, Ts) * x + Bx_Fcn(x, p, u, Ts) * u;
end

function y = h(x, p, u, Ts)
y = ocv_Fcn(x(2)) - u * p(1) - x(1);
end

== matlab function Main/cellStateEstimator/Subsystem/MATLAB Function1 ==
  data: y input; u input; Ts input; x output; s data_store_memory
function x = AF(y, u, Ts)

global s;

%% MAEKF state correction
AEKF_state_correction(y, u, Ts);

s.p = [ Rs_LUT_Fcn(s.x(2)), Rp_LUT_Fcn(s.x(2)), tau_LUT_Fcn(s.x(2)), s.p(4) ]';

%% MAEKF state prediction last
AEKF_state_prediction(y, u, Ts);

x = s.x_;

end

%% State Correction

function AEKF_state_correction(y, u, Ts)

global s;

Cx = Cx_Fcn(s.x_, s.p, u, Ts);

Ex = y - h(s.x_, s.p, u, Ts);
Kx = s.Px_ * Cx' * inv(Cx * s.Px_ * Cx' + s.Rx);
s.x = s.x_ + Kx * Ex;
KCx = Kx * Cx;
s.Px = (eye(size(KCx)) - KCx) * s.Px_;

Hx = cov(s.Ex);

s.lx = uint16(mod(s.lx + 1, s.Lx) + 1);
s.Ex(s.lx) = Ex;

aRx = Hx + Cx * s.Px * Cx';
rx = 0.95;
s.Rx = rx * s.Rx + (1 - rx) * aRx;

aQx = Kx * Hx * Kx';
qx = 0.95;
s.Qx = qx * s.Qx + (1 - qx) * aQx;

end

%% State Prediction

function AEKF_state_prediction(y, u, Ts)

global s

Ax = Ax_Fcn(s.x, s.p, u, Ts);

s.x_ = f(s.x, s.p, u, Ts);
s.Px_ = Ax * s.Px * Ax' + s.Qx;

end

%% OCV and it's derivative with respect to soc (denoted z)

function ocv = ocv_Fcn(z)
g = [-5.90241040764213,13.2176608408928,-6.67518652537707,-2.97531430827542,3.52891506032032,2.99808472821531];

ocv = g(1)*z.^5 + g(2)*z.^4 + g(3)*z.^3 + g(4)*z.^2 + g(5)*z.^1 + g(6);
end

function docv = docv_Fcn(z)
g = [-5.90241040764213,13.2176608408928,-6.67518652537707,-2.97531430827542,3.52891506032032,2.99808472821531];

docv = g(1)*z.^4 + g(2)*z.^3 + g(3)*z.^2 + g(4)*z.^1 + g(5);
end

%% A, B, C, D state matrices

function Ax = Ax_Fcn(x, p, u, Ts)
Ax = [ 
    exp(-Ts / p(3)), 0;
    0, 1
];
end

function Bx = Bx_Fcn(x, p, u, Ts)
Bx = [ 
    (1 - exp(-Ts / p(3))) * p(2);
    Ts / p(4)
];
end

function Cx = Cx_Fcn(x, p, u, Ts)
Cx = [ -1,  docv_Fcn(x(2)) ];
end

function Dx = Dx_Fcn(x, p, u, Ts)
Dx = ocv_Fcn(x(2)) - u * p(1) - x(1) - Cx_Fcn(x, p, u, Ts) * x;
end

%% the F (state transition) and H (measurement) functions

function x_next = f(x, p, u, Ts)
x_next = Ax_Fcn(x, p, u, Ts) * x + Bx_Fcn(x, p, u, Ts) * u;
end

function y = h(x, p, u, Ts)
y = ocv_Fcn(x(2)) - u * p(1) - x(1);
end

%% Parameters LUTS

function Rp = Rp_LUT_Fcn(z)
Rp_LUT = [0.00132849731829051,0.00133071540686515,0.00133106364620441,0.00133282418704394,0.00133927918011939,0.00135371077616641,0.00137940112592065,0.00141963238011775,0.00147768668949337,0.00155684620478314,0.00166039307672272,0.00179160945604776];
soc_LUT = [0,0.0909090909090909,0.181818181818182,0.272727272727273,0.363636363636364,0.454545454545455,0.545454545454545,0.636363636363636,0.727272727272727,0.818181818181818,0.909090909090909,1];

Rp = interp1(soc_LUT, Rp_LUT, z, 'nearest', 'extrap');
end

function Rs = Rs_LUT_Fcn(z)
Rs_LUT = [0.00446224960061823,0.00395928973129493,0.00365723545490869,0.00346135878439388,0.00332839611795259,0.00323577769308545,0.00317057626115591,0.00312485453442757,0.00309346940400882,0.00307294184679812,0.00306083426030356,0.00305538791678206];
soc_LUT = [0,0.0909090909090909,0.181818181818182,0.272727272727273,0.363636363636364,0.454545454545455,0.545454545454545,0.636363636363636,0.727272727272727,0.818181818181818,0.909090909090909,1];

Rs = interp1(soc_LUT, Rs_LUT, z, 'nearest', 'extrap');
end

function tau = tau_LUT_Fcn(z)
tau_LUT = 1000*[0.950871946837005,0.952459545918238,0.952715608141667,0.956801088701637,1.11698000087499,2.16329230815358,2.20434667293784,1.18399583949683,1.06079424954235,1.11432062847071,1.18842633649718,1.28234445639369];
soc_LUT = [0,0.0909090909090909,0.181818181818182,0.272727272727273,0.363636363636364,0.454545454545455,0.545454545454545,0.636363636363636,0.727272727272727,0.818181818181818,0.909090909090909,1];

tau = interp1(soc_LUT, tau_LUT, z, 'nearest', 'extrap');
end
